simulink library "find6DOFSnellMin9_cl"  (R2018b)
settings: Solver=VariableStepAuto  StartTime=0.0  StopTime=10.0  RelTol=1e-3
undefined symbols (not defined in the file or in its folder): params, snells
libraries: powellsMethodMin_ul x1, rayTrace_ul x1
settings Model: Creator=MAE-NCSUCORE  LastModifiedBy=MAE-NCSUCORE

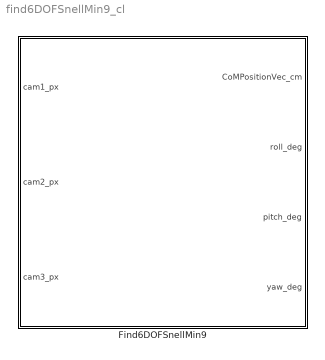
== system find6DOFSnellMin9_cl ==
  Find6DOFSnellMin9 : Subsystem  mask{imageDims_px=params.sideImageSize_px.Value, initialCoMPositionVec_cm=params.initCoMPosVec_cm.Value, initialEulerAngles_deg=params.initEulerAng_deg.Value, indxOfRefVec=params.indexOfRefractionA.Value, glassThickness_cm=params.glassThickness_cm.Value, snells=snells, cameraFOVAngles_deg=params.cameraFOV_deg.Value, sideEulerAngles_deg=params.sideCamEulAng_deg.Value, sideCamPositionVec_cm=params.sideCamPosVec_cm.Value, sideCamDistToGlass_cm=params.sideDistancetoGlass_cm.Value, botEulerAngles_deg=params.botCamEulAng_deg.Value, botCamPositionVec_cm=params.botCamPosVec_cm.Value, botCamDistToGlass_cm=params.botDistancetoGlass_cm.Value, slantEulerAngles_deg=params.slntCamEulAng_deg.Value, slantCamPositionVec_cm=params.slntCamPosVec_cm.Value, slantCamDistToGlass_cm=params.slntDistancetoGlass_cm.Value, sideSeparation_cm=params.sideDotSepDist_cm.Value, sidePositionVecBF_cm=params.sideDotPosVec_cm.Value, bottomASeparation_cm=params.botADotSepDist_cm.Value, botAPositionVecBF_cm=params.botADotPosVec_cm.Value, bottomBSeparation_cm=params.botBDotSepDist_cm.Value, botBPositionVecBF_cm=params.botBDotPosVec_cm.Value}
      mask prompts: imageDims_px "Image Dimensions [rows, cols] [px]"; initialCoMPositionVec_cm "Initial CoM Position Vector [cm]"; initialEulerAngles_deg "Initial Euler Angles [deg]"; indxOfRefVec "Indices of Refraction, [air glass water]"; glassThickness_cm "Glass Thickness [cm]"; snells "Snells Parameter Structure"; cameraFOVAngles_deg "Field of View Angles [horiz, vert] [deg]"; sideEulerAngles_deg "Euler Angles [roll pitch yaw] [deg]"; sideCamPositionVec_cm "Position Vector [cm]"; sideCamDistToGlass_cm "Distance to Glass [cm]"; botEulerAngles_deg "Euler Angles [roll pitch yaw]  [deg]"; botCamPositionVec_cm "Position Vector [cm]"; botCamDistToGlass_cm "Distance to Glass [cm]"; slantEulerAngles_deg "Euler Angles [roll pitch yaw]  [deg]"; slantCamPositionVec_cm "Position Vec [cm]"; slantCamDistToGlass_cm "Distance to Glass [cm]"; sideSeparation_cm "Separation Distance [cm]"; sidePositionVecBF_cm "Centroid Position in Body Frame [cm]"; bottomASeparation_cm "Separation Distance [cm]"; botAPositionVecBF_cm "Centroid Position in Body Frame [cm]"; bottomBSeparation_cm "Separation Distance [cm]"; botBPositionVecBF_cm "Centroid Position in Body Frame [cm]"
      mask init:
      | find6DOFSnellMin_init;
      mask DialogControl Container4 Prompt: Camera Properties
      mask DialogControl Container7 Prompt: Side Camera
      mask DialogControl Container8 Prompt: Bottom Camera
      mask DialogControl Container9 Prompt: Slant Camera
      mask DialogControl Container13 Prompt: Dot Properties
      mask DialogControl Container14 Prompt: Side Dots
      mask DialogControl Container15 Prompt: Bottom Dot Set A
      mask DialogControl Container16 Prompt: Bottom Dot Set B
      mask Display:
      | image('blockImage.png',[.2, .2, .6, .6],'on');
      | 
      | port_label('input',1,'Camera 1')
      | port_label('input',2,'Camera 2')
      | port_label('input',3,'Camera 3')
      | 
      | port_label('output',1,'CoMPosVec_cm')
      | port_label('output',2,'roll_rad')
      | port_label('output',3,'pitch_rad')
      | port_label('output',4,'yaw_rad')
      | 
      | % port_label('output',4,'err')
      | % port_label('output',5,'rxRaw')
      | % port_label('output',6,'ryRaw')
      | 
      | text(0.5, 1, 'Snells Law - Resolve 6 DOF', 'horizontalAlignment', 'center', ...
      |   'verticalAlignment', 'top')

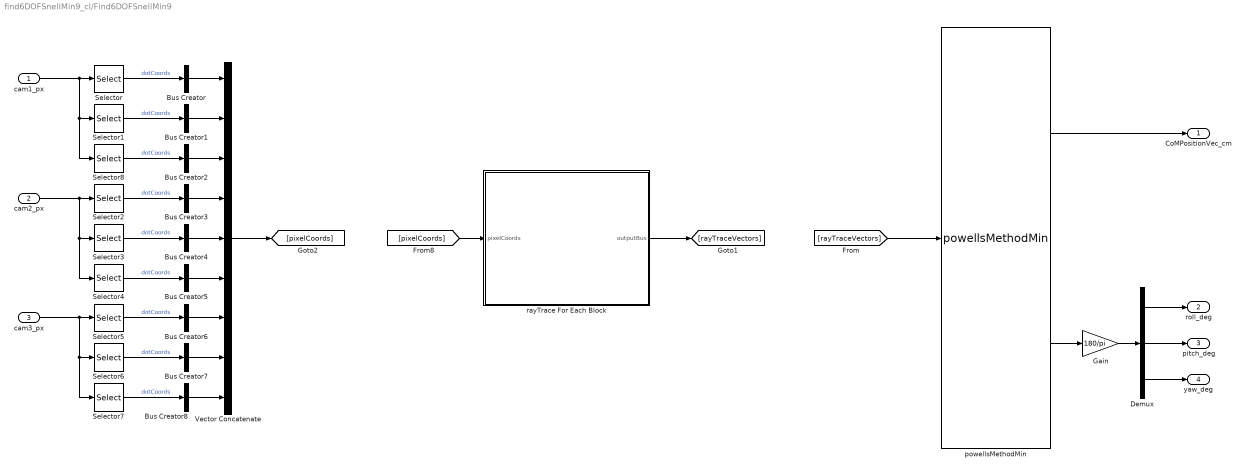
== system find6DOFSnellMin9_cl/Find6DOFSnellMin9 ==
  cam1_px : Inport
  cam2_px : Inport  Port=2
  cam3_px : Inport  Port=3
  Bus Creator{,1..8} (9 alike) : BusCreator  Inputs=1  OutDataTypeStr=Bus: coordBus  NonVirtualBus=on
  Demux : Demux  Outputs=3
  Gain : Gain  Gain=180/pi
  Selector : Selector  InputPortWidth=6  IndexOptions=Index vector (dialog)  Indices=[1 2]  OutputSizes=1
  Selector1 : Selector  InputPortWidth=6  IndexOptions=Index vector (dialog)  Indices=[3 4]  OutputSizes=1
  Selector2 : Selector  InputPortWidth=6  IndexOptions=Index vector (dialog)  Indices=[1 2]  OutputSizes=1
  Selector3 : Selector  InputPortWidth=6  IndexOptions=Index vector (dialog)  Indices=[3 4]  OutputSizes=1
  Selector4 : Selector  InputPortWidth=6  IndexOptions=Index vector (dialog)  Indices=[5 6]  OutputSizes=1
  Selector5 : Selector  InputPortWidth=6  IndexOptions=Index vector (dialog)  Indices=[1 2]  OutputSizes=1
  Selector6 : Selector  InputPortWidth=6  IndexOptions=Index vector (dialog)  Indices=[3 4]  OutputSizes=1
  Selector7 : Selector  InputPortWidth=6  IndexOptions=Index vector (dialog)  Indices=[5 6]  OutputSizes=1
  Selector8 : Selector  InputPortWidth=6  IndexOptions=Index vector (dialog)  Indices=[5 6]  OutputSizes=1
  Vector Concatenate : Concatenate  NumInputs=9
  powellsMethodMin : powellsMethodMin_ul/powellsMethodMin  initialEulerAngles_rad=initialEulerAngles_rad  snells=snells
  rayTrace For Each Block : Subsystem  TreatAsAtomicUnit=on  mask{camPosVec_cm=snells.camPosVec, camEulerAngles_deg=snells.camEulAng, dist2Glass_cm=snells.camDist2Glass, indOfReFVec=indxOfRefVec, glassPlane=2, glassThickness_cm=glassThickness_cm, imageDimsVec_px=imageDims_px, camFOV_deg=cameraFOVAngles_deg}
      mask prompts: camPosVec_cm "Camera Position Vector [cm]"; camEulerAngles_deg "Camera Euler Angles [deg]"; dist2Glass_cm "Distance to Glass [cm]"; indOfReFVec "Indices of Refraction [air glass water]"; glassPlane "Glass Plane (1 = xy, 2 = xz)"; glassThickness_cm "Glass Thickness [cm]"; imageDimsVec_px "Image Dimensions [px], [rows cols]"; camFOV_deg "Camera Field of View [deg], [horiz vert]"
  CoMPositionVec_cm : Outport
  roll_deg : Outport  Port=2
  pitch_deg : Outport  Port=3
  yaw_deg : Outport  Port=4
  wires:
  Selector/1 -> Bus Creator/1  "dotCoords"
  Selector1/1 -> Bus Creator1/1  "dotCoords"
  powellsMethodMin/1 -> CoMPositionVec_cm/1
  powellsMethodMin/2 -> Gain/1
  Gain/1 -> Demux/1
  Demux/1 -> roll_deg/1
  Demux/3 -> yaw_deg/1
  Demux/2 -> pitch_deg/1
  cam1_px/1 -> Selector/1, Selector1/1, Selector8/1
  Selector8/1 -> Bus Creator2/1  "dotCoords"
  Selector4/1 -> Bus Creator5/1  "dotCoords"
  cam2_px/1 -> Selector4/1, Selector3/1, Selector2/1
  Selector3/1 -> Bus Creator4/1  "dotCoords"
  Selector2/1 -> Bus Creator3/1  "dotCoords"
  Selector5/1 -> Bus Creator6/1  "dotCoords"
  Selector6/1 -> Bus Creator7/1  "dotCoords"
  cam3_px/1 -> Selector5/1, Selector6/1, Selector7/1
  Selector7/1 -> Bus Creator8/1  "dotCoords"
  Bus Creator1/1 -> Vector Concatenate/2
  Bus Creator/1 -> Vector Concatenate/1
  Bus Creator2/1 -> Vector Concatenate/3
  Bus Creator3/1 -> Vector Concatenate/4
  Bus Creator4/1 -> Vector Concatenate/5
  Bus Creator5/1 -> Vector Concatenate/6
  Bus Creator6/1 -> Vector Concatenate/7
  Bus Creator7/1 -> Vector Concatenate/8
  Bus Creator8/1 -> Vector Concatenate/9
  Vector Concatenate/1 -> [pixelCoords]
  [pixelCoords] -> rayTrace For Each Block/1(pixelCoords)
  rayTrace For Each Block/1(outputBus) -> [rayTraceVectors]
  [rayTraceVectors] -> powellsMethodMin/1

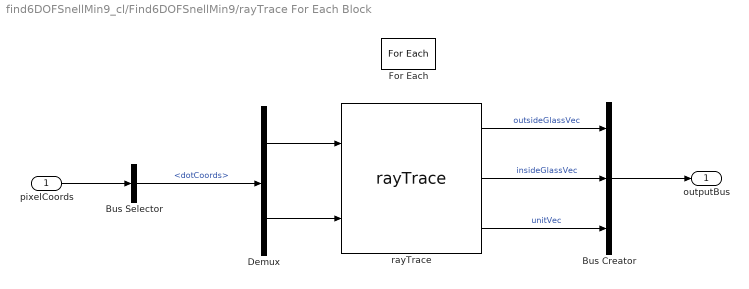
== system find6DOFSnellMin9_cl/Find6DOFSnellMin9/rayTrace For Each Block ==
  pixelCoords : Inport  Partition=on  PartitionDimension=1  PartitionWidth=1  PartitionOffset=0
  Bus Creator : BusCreator  Inputs=3  OutDataTypeStr=Bus: rayBus  NonVirtualBus=on
  Bus Selector : BusSelector  OutputSignals=dotCoords
  Demux : Demux  Outputs=2
  For Each : ForEach  DisableCoverage=on  IterateSubsysMaskParameter=on,on,on,off,off,off,off,off  IndexMode=One-based
  rayTrace : rayTrace_ul/rayTrace  camPosVec_cm=botCamPositionVec_cm  camEulAngles_deg=botEulerAngles_deg  dist2Glass_cm=botCamDistToGlass_cm  indOfRefVec=indxOfRefVec  glassPlane=1  glassThickness_cm=glassThickness_cm  imageDimsVec_px=imageDims_px  camFOV_deg=cameraFOVAngles_deg
  outputBus : Outport  ConcatenationDimension=1
  wires:
  Demux/2 -> rayTrace/2
  Demux/1 -> rayTrace/1
  rayTrace/1 -> Bus Creator/1  "outsideGlassVec"
  pixelCoords/1 -> Bus Selector/1
  Bus Selector/1 -> Demux/1  "<dotCoords>"
  Bus Creator/1 -> outputBus/1
  rayTrace/2 -> Bus Creator/2  "insideGlassVec"
  rayTrace/3 -> Bus Creator/3  "unitVec"
